simulink model "UNIFIER"  (R2023b)
settings: Solver=ode1  StartTime=0.0  StopTime=194  FixedStep=1/500  RelTol=1e-3
values from neighbouring files (symbols this model uses):
  b = 20.11467    [UNIFIERLanding_20240613_190735.mat]    (also in UNIFIER_LOAD.m; UNIFIER_LOADsim.m; UNIFIER_trim_out_20240612_032607.mat)
  c = 1.43676    [UNIFIERLanding_20240613_190735.mat]    (also in UNIFIER_LOAD.m; UNIFIER_LOADsim.m; UNIFIER_trim_out_20240612_032607.mat)
  DEP_INTEG_IC = 117.49388    [UNIFIER_LOAD.m]    (also in UNIFIER_LOADsim.m; UNIFIER_trim_out_20240612_032607.mat)
  dp_DEP =     [UNIFIERLanding_20240613_190735.mat]    (also in UNIFIER_trim_out_20240612_032607.mat)
  dp_FUSE_FIN =     [UNIFIER_trim_out_20240612_032607.mat]
  dp_HTU =     [UNIFIERLanding_20240613_190735.mat]    (also in UNIFIER_trim_out_20240612_032607.mat)
  dp_VTAIL =     [UNIFIER_trim_out_20240612_032607.mat]
  dp_VTAIL_INDUCED =     [UNIFIER_trim_out_20240612_032607.mat]
  dp_WING_root =     [UNIFIER_trim_out_20240612_032607.mat]
  dp_WING_tip =     [UNIFIER_trim_out_20240612_032607.mat]
  dumax = [1.0471975512 1.0471975512 1.0471975512 0.174532925199 2 2 2]    [UNIFIERLanding_20240613_190735.mat]
  Euler0 = xstar(7:9)'    [UNIFIER_6DOFsim_init.m]    (also in UNIFIER_LOAD.m = [0, 0, 0]; UNIFIER_LOADsim.m = [0, 0, 0]; UNIFIER_trim_out_20240612_032607.mat = [3.43106170069e-06 0.0515008506278 -2.79252663434])
  ground_alt = 0    [UNIFIER_LOAD.m]    (also in UNIFIER_LOADsim.m; UNIFIER_trim_out_20240612_032607.mat)
  m = 7057    [UNIFIERLanding_20240613_190735.mat]    (also in UNIFIER_LOAD.m; UNIFIER_LOADsim.m; UNIFIER_trim_out_20240612_032607.mat)
  omegab0 = xstar(10:12)'    [UNIFIER_6DOFsim_init.m]    (also in UNIFIER_LOAD.m = [0,0,0]; UNIFIER_LOADsim.m = [0,0,0]; UNIFIER_trim_out_20240612_032607.mat = [0 0 0])
  S = 29.98388    [UNIFIERLanding_20240613_190735.mat]    (also in UNIFIER_LOAD.m; UNIFIER_LOADsim.m; UNIFIER_trim_out_20240612_032607.mat)
  sensor_delay_steps = 5    [UNIFIER_LOAD.m]    (also in UNIFIER_LOADsim.m; UNIFIER_trim_out_20240612_032607.mat)
  solution =     [UNIFIERLanding_20240613_190735.mat]
  u1_0 = [ustar(1), -1*ustar(1), ustar(3)-ustar(2), ustar(3)+ustar(2), ustar(4), ustar(4)]    [UNIFIER_6DOFsim_init.m]    (also in UNIFIER_LOAD.m = [2.1112539e-05, -2.1112539e-05, -0.085004635, -0.084972650, ; UNIFIER_LOADsim.m = [2.1112539e-05, -2.1112539e-05, -0.085004635, -0.084972650, ; UNIFIER_trim_out_20240612_032607.mat = [2.1112539e-05 -2.1112539e-05 -0.085004635 -0.08497265 0.197)
  u2_0 = ones(1,12) .* ustar(5)    [UNIFIER_6DOFsim_init.m]    (also in UNIFIER_LOAD.m = ones(1,12) .* 0.4252; UNIFIER_LOADsim.m = ones(1,12) .* 0.4252; UNIFIER_trim_out_20240612_032607.mat = [0.4252 0.4252 0.4252 0.4252 0.4252 0.4252 0.4252 0.4252 0.4)
  u3_0 = ustar(7)    [UNIFIER_6DOFsim_init.m]    (also in UNIFIER_LOAD.m = 0.089689; UNIFIER_LOADsim.m = 0.089689; UNIFIER_trim_out_20240612_032607.mat = 0.089689)
  u4_0 = 0    [UNIFIER_6DOFsim_init.m]    (also in UNIFIER_LOAD.m; UNIFIER_LOADsim.m; UNIFIER_trim_out_20240612_032607.mat)
  u_trim = ustar    [UNIFIER_6DOFsim_init.m]    (also in UNIFIER_LOAD.m = [0.0; UNIFIER_LOADsim.m = [0.0)
  umax = [0.436332312999 0.523598775598 0.523598775598 0.436332312999 1 1 1]    [UNIFIERLanding_20240613_190735.mat]    (also in UNIFIER_trim_out_20240612_032607.mat)
  umin = [-0.436332312999 -0.523598775598 -0.523598775598 0 0 -1 -0.5]    [UNIFIERLanding_20240613_190735.mat]    (also in UNIFIER_trim_out_20240612_032607.mat)
  Va = [72.7399985115 72.2978466179 70.3592089076 68.5755686022 67.5674222915 66.8967003826 65.8958642605 64.4243196248 62.667507398 61.0171213882 59.8601734245 59.2796795419 ... (250 elements, 250x1)]    [UNIFIERLanding_20240613_190735.mat]
  Vb0 = xstar(4:6)'    [UNIFIER_6DOFsim_init.m]    (also in UNIFIER_LOAD.m = [72.731047032614440, 0, 1.142307104518741]; UNIFIER_LOADsim.m = [72.731047032614440, 0, 1.142307104518741]; UNIFIER_trim_out_20240612_032607.mat = [52.6789583502 0 2.71559652634])
  vtail_dist_to_wing = 7.8070    (= 7.807)    [UNIFIER_LOAD.m]    (also in UNIFIER_LOADsim.m; UNIFIER_trim_out_20240612_032607.mat)
  vtail_nodes = [dp_VTAIL.Xs_LE;     dp_VTAIL.Ys_LE;     dp_VTAIL.Zs_LE]    [UNIFIER_LOAD.m]    (also in UNIFIER_LOADsim.m; UNIFIER_trim_out_20240612_032607.mat = [-16.4894695282 -2.83441376686 -2.73765826225 -16.1370849609)
  wing_nodes = [fliplr(dp_WING_tip.LE_Xs),fliplr(dp_WING_root.LE_Xs),dp_WING_root.LE_Xs,dp_WING_tip.LE_Xs;     fliplr(-dp_WING_tip.LE_Ys),fliplr(-dp_WING_root.LE_Ys),dp_WING_root.LE_Ys,dp_WING_tip.LE_Ys;     fliplr(dp_WING_tip.LE_Zs),fliplr(dp_WING_root.LE_Zs),dp_WING_root.LE_Zs,dp_WING_tip.LE_Zs]    [UNIFIER_LOAD.m]    (also in UNIFIER_LOADsim.m; UNIFIER_trim_out_20240612_032607.mat = [-7.70795631409 -9.67500019073 -0.98178178072 -7.66801691055)
  Xe0 = xstar(1:3)'    [UNIFIER_6DOFsim_init.m]    (also in UNIFIER_LOAD.m = [0,0,-1219]; UNIFIER_LOADsim.m = [0,0,-1219]; UNIFIER_trim_out_20240612_032607.mat = [0 0 -1100])
  xyz_cg = [-8.09 0 -0.2]    [UNIFIERLanding_20240613_190735.mat]    (also in UNIFIER_LOAD.m = [-8.09,0,-0.2]; UNIFIER_LOADsim.m = [-8.09,0,-0.2]; UNIFIER_trim_out_20240612_032607.mat)
  xyz_DEP = [-6.9629998 -10.05 -0.90899998 -6.921 -8.4499998 -0.792 -6.8660002 -6.8499999 -0.82300001 -6.8099999 -5.25 -0.85000002 ... (36 elements, 3x12)]    [UNIFIERLanding_20240613_190735.mat]    (also in UNIFIER_LOAD.m = [ -6.9629998	-6.9210000	-6.8660002	-6.8099999	-6.7540002	-6.; UNIFIER_LOADsim.m = [ -6.9629998	-6.9210000	-6.8660002	-6.8099999	-6.7540002	-6.; UNIFIER_trim_out_20240612_032607.mat)
undefined symbols (not defined in the file or in its folder): Earth, F, MIL, WGS84
libraries: simulink_extras x23, aerolibactuator x16, dspnetwork x15, sharedutil x14, sharedtransform x7, aerolibtransform2 x5, slpidlib x5, simulink x5, aerolibwind2 x4, matrix_library x1, shared6dof x1, aerolibatmos2 x1
(part 4 of 6)

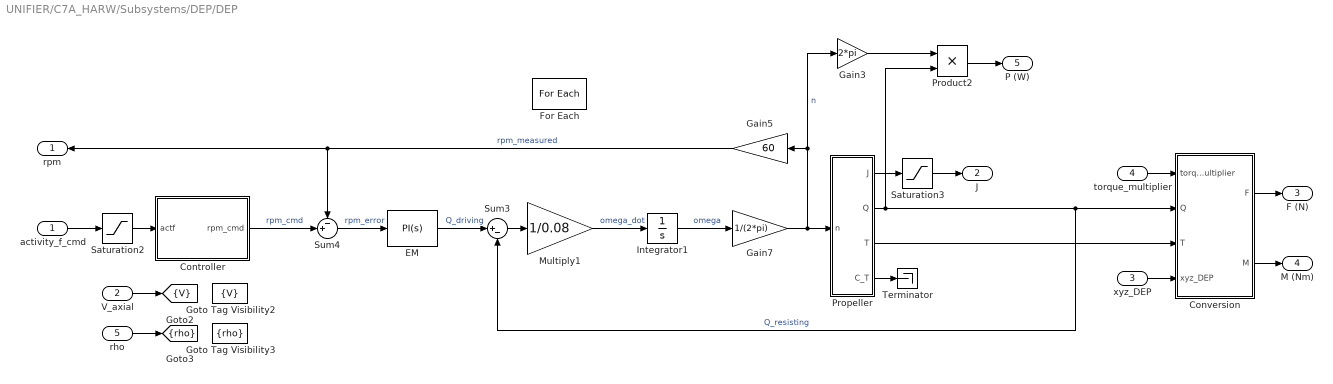
== system UNIFIER/C7A_HARW/Subsystems/DEP/DEP ==
  activity_f_cmd : Inport  Partition=on  PartitionDimension=1  PartitionWidth=1  PartitionOffset=0
  V_axial : Inport  Port=2  Partition=on  PartitionDimension=1  PartitionWidth=1  PartitionOffset=0
  xyz_DEP : Inport  Port=3  Partition=on  PartitionDimension=2  PartitionWidth=1  PartitionOffset=0
  torque_multiplier : Inport  Port=4  Partition=on  PartitionDimension=1  PartitionWidth=1  PartitionOffset=0
  rho : Inport  Port=5
  Controller : Subsystem
  Conversion : Subsystem
  EM : slpidlib/PID Controller  Controller=PI  Form=Parallel  TimeDomain=Continuous-time  UseExternalTs=off  SampleTime=-1  IntegratorMethod=Forward Euler  FilterMethod=Forward Euler  ControllerParametersSource=internal  P=0.768856317292492  I=33.2713838828509  UseKiTs=off  D=0  N=100  UseFilter=on  TunerSelectOption=Transfer Function Based (PID Tuner App)  InitialConditionSource=internal  InitialConditionForIntegrator=DEP_PID_IC  InitialConditionForFilter=0  DifferentiatorICPrevScaledInput=0  ExternalReset=none  TrackingMode=off  Kt=1  LimitOutput=on  SatLimitsSource=internal  UpperSaturationLimit=284  LowerSaturationLimit=-284  LinearizeAsGain=on  AntiWindupMode=clamping  Kb=1  LimitIntegrator=off  UpperIntegratorSaturationLimit=inf  LowerIntegratorSaturationLimit=-inf  POutMin=[]  POutMax=[]  IOutMin=[]  IOutMax=[]  DOutMin=[]  DOutMax=[]  NOutMin=[]  NOutMax=[]  SumOutMin=[]  SumOutMax=[]  SaturationOutMin=[]  SaturationOutMax=[]  PParamMin=[]  PParamMax=[]  IParamMin=[]  IParamMax=[]  DParamMin=[]  DParamMax=[]  NParamMin=[]  NParamMax=[]  KbParamMin=[]  KbParamMax=[]  KtParamMin=[]  KtParamMax=[]  KbOutMin=[]  KbOutMax=[]  KtOutMin=[]  KtOutMax=[]  IntegratorOutMin=[]  IntegratorOutMax=[]  FilterOutMin=[]  FilterOutMax=[]  SumI1OutMin=[]  SumI1OutMax=[]  SumI2OutMin=[]  SumI2OutMax=[]  SumI3OutMin=[]  SumI3OutMax=[]  SumI4OutMin=[]  SumI4OutMax=[]  SumDOutMin=[]  SumDOutMax=[]  DifferentiatorOutMin=[]  DifferentiatorOutMax=[]  FilterDiffOutCoefMin=[]  FilterDiffOutCoefMax=[]  ReciprocalOutMin=[]  ReciprocalOutMax=[]  SumDenOutMin=[]  SumDenOutMax=[]  SumNumOutMin=[]  SumNumOutMax=[]  DivideOutMin=[]  DivideOutMax=[]  UdiffTsProdOutMin=[]  UdiffTsProdOutMax=[]  NTsProdOutMin=[]  NTsProdOutMax=[]  UintegralTsProdOutMin=[]  UintegralTsProdOutMax=[]  UngainTsProdOutMin=[]  UngainTsProdOutMax=[]  ClampingZeroOutDataTypeStr=Inherit: Inherit via back propagation  ClampingZeroOutMin=[]  ClampingZeroOutMax=[]  FilterDenConstantOutDataTypeStr=Inherit: Inherit via back propagation  FilterDenConstantOutMin=[]  FilterDenConstantOutMax=[]  PCopyOutDataTypeStr=Inherit: Inherit via back propagation  PCopyOutMin=[]  PCopyOutMax=[]  NCopyOutDataTypeStr=Inherit: Inherit via back propagation  NCopyOutMin=[]  NCopyOutMax=[]  IntegratorContinuousStateAttributes=''  IntegratorStateMustResolveToSignalObject=off  IntegratorRTWStateStorageClass=Auto  FilterContinuousStateAttributes=''  FilterStateMustResolveToSignalObject=off  FilterRTWStateStorageClass=Auto  ParallelPVariant=InternalParameters  IdealPVariant=Disabled  IVariant=InternalParameters  DVariant=Disabled  IntegratorVariant=Continuous  SatVariant=Enabled  AWVariant=ContClampingParallel  PCopyVariant=Disabled  TRVariant=Disabled  FdbkBlocksVariant=Forward  IdealPFdbkVariant=Disabled  SatFdbkVariant=Disabled  DerivativeFilterVariant=Disabled  NVariant=Disabled  NCopyVariant=Disabled_SignalSpec  FilterICVariant=Disabled  IntegratorICVariant=InternalICs  ExternalResetVariant=Disabled  TRSumVariant=Passthrough  SumFdbkVariant=Disabled  SumVariant=Sum_PI  TsampFilterVariant=InternalTs  TsampNgainVariant=Passthrough  TsampIntegralVariant=Disabled_SignalSpec  ExternalSaturationOutDataTypeStr=Inherit: Same as second input
  For Each : ForEach  DisableCoverage=on  SpecifiedNumIters=12
  Gain3 : Gain  Gain=2*pi
  Gain5 : Gain  Gain=60
  Gain7 : Gain  Gain=1/(2*pi)
  Goto Tag Visibility2 : GotoTagVisibility  GotoTag=V
  Goto Tag Visibility3 : GotoTagVisibility  GotoTag=rho
  Integrator1 : Integrator  InitialCondition=DEP_INTEG_IC
  Multiply1 : Gain  Gain=1/0.08
  Product2 : Product
  Propeller : Subsystem
  Saturation2 : Saturate  UpperLimit=1  LowerLimit=0
  Saturation3 : Saturate  UpperLimit=5  LowerLimit=0.2
  Sum3 : Sum  Inputs=|+-
  Sum4 : Sum  Inputs=-+|
  Terminator : Terminator
  rpm : Outport  ConcatenationDimension=1
  J : Outport  Port=2  ConcatenationDimension=1
  F (N) : Outport  Port=3  ConcatenationDimension=2
  M (Nm) : Outport  Port=4  ConcatenationDimension=2
  P (W) : Outport  Port=5  ConcatenationDimension=1
  tag scope: V=scoped, rho=scoped
  wires:
  Conversion/1(F) -> F (N)/1
  Conversion/2(M) -> M (Nm)/1
  Saturation3/1 -> J/1
  Propeller/4(C_T) -> Terminator/1
  activity_f_cmd/1 -> Saturation2/1
  Propeller/1(J) -> Saturation3/1
  Controller/1(rpm_cmd) -> Sum4/2  "rpm_cmd"
  Gain3/1 -> Product2/1
  xyz_DEP/1 -> Conversion/4(xyz_DEP)
  Multiply1/1 -> Integrator1/1  "omega_dot"
  Sum4/1 -> EM/1  "rpm_error"
  Gain7/1 -> Gain3/1, Gain5/1, Propeller/1(n)  "n"
  EM/1 -> Sum3/1  "Q_driving"
  V_axial/1 -> [V]
  Product2/1 -> P (W)/1
  torque_multiplier/1 -> Conversion/1(torque_multiplier)
  Gain5/1 -> rpm/1, Sum4/1  "rpm_measured"
  Propeller/3(T) -> Conversion/3(T)
  rho/1 -> [rho]
  Propeller/2(Q) -> Product2/2, Conversion/2(Q), Sum3/2  "Q_resisting"
  Saturation2/1 -> Controller/1(actf)
  Sum3/1 -> Multiply1/1
  Integrator1/1 -> Gain7/1  "omega"

== system UNIFIER/C7A_HARW/Subsystems/HTU/PropAndMotor ==
  Vrw_mag_eas : Inport
  T_cmd (N) : Inport  Port=2
  1-D Lookup Table : Lookup_n-D  NumberOfTableDimensions=1  BreakpointsForDimension1=dp_HTU.limits.V_low_lim  IndexSearchMethod=Linear search  BeginIndexSearchUsingPreviousIndexResult=on  Table=dp_HTU.limits.T_low_lim  InternalRulePriority=Speed  RndMeth=Simplest
  1-D Lookup Table1 : Lookup_n-D  NumberOfTableDimensions=1  BreakpointsForDimension1=dp_HTU.limits.V_up_lim  IndexSearchMethod=Linear search  BeginIndexSearchUsingPreviousIndexResult=on  Table=dp_HTU.limits.T_up_lim  InternalRulePriority=Speed  RndMeth=Simplest
  Linear Second-Order Actuator : aerolibactuator/Linear Second-Order Actuator  wn_fin=8  z_fin=1.1  fin_act_0=0  fin_act_vel=0
  P lookup : Lookup_n-D  BreakpointsForDimension1=dp_HTU.V_vec  BreakpointsForDimension2=dp_HTU.T_vec  IndexSearchMethod=Linear search  BeginIndexSearchUsingPreviousIndexResult=on  Table=dp_HTU.P_grid  InternalRulePriority=Speed  RndMeth=Simplest
      settings: InputPortMap=u0,u1
  Saturation Dynamic : simulink/Discontinuities/Saturation Dynamic  OutMin=[]  OutMax=[]  OutDataTypeStr=Inherit: Same as second input  OutDataType=fixdt(1, 16)  OutScaling=2^-10  DoSatur=off
  P (kW) : Outport
  T (N) : Outport  Port=2
  wires:
  Vrw_mag_eas/1 -> P lookup/1, 1-D Lookup Table/1, 1-D Lookup Table1/1
  Saturation Dynamic/1 -> Linear Second-Order Actuator/1
  P lookup/1 -> P (kW)/1
  1-D Lookup Table1/1 -> Saturation Dynamic/1
  1-D Lookup Table/1 -> Saturation Dynamic/3
  T_cmd (N)/1 -> Saturation Dynamic/2
  Linear Second-Order Actuator/1 -> T (N)/1, P lookup/2

== system UNIFIER/C7A_HARW/Subsystems/LandingGears/LeftMain ==
  xyz_gear : Inport  PortDimensions=3
  Euler : Inport  Port=2  PortDimensions=3
  X_e : Inport  Port=3  PortDimensions=3
  ground_alt : Inport  Port=4
  omega : Inport  Port=5
  V_b : Inport  Port=6  PortDimensions=3
  DetermineGroundImpact : Subsystem
  FrameTransfer : Subsystem
  GearForceSystem : Subsystem
      settings: PortSchema="{\"entries\":[{\"content\":{\"sides\":[{\"content\":{\"connectorIds\":[\"In1\",\"In2\"]},\"type\":\"ConnectorPlacement.EquallySpacedRectSide\",\"uuid\":\"d290905f-60cf-4bc0-bab1-4e61329254ed\"},{\"content\":{\"connectorIds\":[\"Out1\"],\"side\":\"RIGHT\"},\"type\":\"ConnectorPlacement.EquallySpacedRectSide\",\"uuid\":\"8978d452-e293-46ff-9875-eaa6c076b0ed\"},{\"content\":{\"connectorIds\":[\"In3\"],\"side\":\"TOP\"},\"type\":\"ConnectorPlacement.EquallySpacedRectSide\",\"uuid\":\"a7915404-bc15-4a50-b2f6-71702d493273\"},{\"content\":{\"connectorIds\":[],\"side\":\"HIDDEN\"},\"type\":\"ConnectorPlacement.EquallySpacedRectSide\",\"uuid\":\"71da3c07-875d-44a9-a817-88149ba8aea4\"}]},\"type\":\"ConnectorPlacement.EquallySpacedConnector\",\"uuid\":\"ffb36ab3-c4a0-4dd1-8d55-bd9c51a110f4\"}],\"packageUris\":[\"http://schema.mathworks.com/mf0/Connector/R2020b\"],\"version\":\"1.0\"}"
  GetDeflection : Subsystem
  PointAndVelocityTransformation : Subsystem
  Scope : Scope
  Scope1 : Scope
  Scope3 : Scope
  F : Outport
  M : Outport  Port=2
  impact_flag : Outport  Port=3
  wires:
  DetermineGroundImpact/1(dz_to_ground) -> Scope/1
  ground_alt/1 -> DetermineGroundImpact/2(ground_alt)
  GetDeflection/1(dz) -> GearForceSystem/2(dz)
  PointAndVelocityTransformation/1(X_gear) -> GetDeflection/2(X_tip), DetermineGroundImpact/1(X_gear)
  GearForceSystem/1(F_gear_total) -> Scope1/1, FrameTransfer/2(F_gear_total)
  omega/1 -> PointAndVelocityTransformation/4(omega)
  xyz_gear/1 -> PointAndVelocityTransformation/1(xyz_gear), FrameTransfer/1(xyz_shock_absorber)
  FrameTransfer/2(M_b) -> M/1
  DetermineGroundImpact/2(impact_flag) -> impact_flag/1, GearForceSystem/3(impact_flag), Scope3/1
  V_b/1 -> PointAndVelocityTransformation/5(V_b)
  FrameTransfer/1(F_b) -> F/1
  DetermineGroundImpact/3(X_impact) -> GetDeflection/1(X_impact)
  PointAndVelocityTransformation/2(V_gear) -> GearForceSystem/1(V_gear)
  X_e/1 -> PointAndVelocityTransformation/2(X_e)
  Euler/1 -> PointAndVelocityTransformation/3(Euler)

== system UNIFIER/C7A_HARW/Subsystems/LandingGears/Nose ==
  xyz_gear : Inport  PortDimensions=3
  Euler : Inport  Port=2  PortDimensions=3
  X_e : Inport  Port=3  PortDimensions=3
  ground_alt : Inport  Port=4
  omega : Inport  Port=5
  V_b : Inport  Port=6  PortDimensions=3
  DetermineGroundImpact : Subsystem
  FrameTransfer : Subsystem
  GearForceSystem : Subsystem
      settings: PortSchema="{\"entries\":[{\"content\":{\"sides\":[{\"content\":{\"connectorIds\":[\"In1\",\"In2\"]},\"type\":\"ConnectorPlacement.EquallySpacedRectSide\",\"uuid\":\"d290905f-60cf-4bc0-bab1-4e61329254ed\"},{\"content\":{\"connectorIds\":[\"Out1\"],\"side\":\"RIGHT\"},\"type\":\"ConnectorPlacement.EquallySpacedRectSide\",\"uuid\":\"8978d452-e293-46ff-9875-eaa6c076b0ed\"},{\"content\":{\"connectorIds\":[\"In3\"],\"side\":\"TOP\"},\"type\":\"ConnectorPlacement.EquallySpacedRectSide\",\"uuid\":\"a7915404-bc15-4a50-b2f6-71702d493273\"},{\"content\":{\"connectorIds\":[],\"side\":\"HIDDEN\"},\"type\":\"ConnectorPlacement.EquallySpacedRectSide\",\"uuid\":\"71da3c07-875d-44a9-a817-88149ba8aea4\"}]},\"type\":\"ConnectorPlacement.EquallySpacedConnector\",\"uuid\":\"ffb36ab3-c4a0-4dd1-8d55-bd9c51a110f4\"}],\"packageUris\":[\"http://schema.mathworks.com/mf0/Connector/R2020b\"],\"version\":\"1.0\"}"
  GetDeflection : Subsystem
  PointAndVelocityTransformation : Subsystem
  Scope : Scope
  Scope1 : Scope
  Scope3 : Scope
  F : Outport
  M : Outport  Port=2
  impact_flag : Outport  Port=3
  wires:
  DetermineGroundImpact/1(dz_to_ground) -> Scope/1
  ground_alt/1 -> DetermineGroundImpact/2(ground_alt)
  GetDeflection/1(dz) -> GearForceSystem/2(dz)
  PointAndVelocityTransformation/1(X_gear) -> GetDeflection/2(X_tip), DetermineGroundImpact/1(X_gear)
  GearForceSystem/1(F_gear_total) -> Scope1/1, FrameTransfer/2(F_gear_total)
  omega/1 -> PointAndVelocityTransformation/4(omega)
  xyz_gear/1 -> PointAndVelocityTransformation/1(xyz_gear), FrameTransfer/1(xyz_shock_absorber)
  FrameTransfer/2(M_b) -> M/1
  DetermineGroundImpact/2(impact_flag) -> impact_flag/1, GearForceSystem/3(impact_flag), Scope3/1
  V_b/1 -> PointAndVelocityTransformation/5(V_b)
  FrameTransfer/1(F_b) -> F/1
  DetermineGroundImpact/3(X_impact) -> GetDeflection/1(X_impact)
  PointAndVelocityTransformation/2(V_gear) -> GearForceSystem/1(V_gear)
  X_e/1 -> PointAndVelocityTransformation/2(X_e)
  Euler/1 -> PointAndVelocityTransformation/3(Euler)

== system UNIFIER/C7A_HARW/Subsystems/LandingGears/RightMain ==
  xyz_gear : Inport  PortDimensions=3
  Euler : Inport  Port=2  PortDimensions=3
  X_e : Inport  Port=3  PortDimensions=3
  ground_alt : Inport  Port=4
  omega : Inport  Port=5
  V_b : Inport  Port=6  PortDimensions=3
  DetermineGroundImpact : Subsystem
  FrameTransfer : Subsystem
  GearForceSystem : Subsystem
      settings: PortSchema="{\"entries\":[{\"content\":{\"sides\":[{\"content\":{\"connectorIds\":[\"In1\",\"In2\"]},\"type\":\"ConnectorPlacement.EquallySpacedRectSide\",\"uuid\":\"d290905f-60cf-4bc0-bab1-4e61329254ed\"},{\"content\":{\"connectorIds\":[\"Out1\"],\"side\":\"RIGHT\"},\"type\":\"ConnectorPlacement.EquallySpacedRectSide\",\"uuid\":\"8978d452-e293-46ff-9875-eaa6c076b0ed\"},{\"content\":{\"connectorIds\":[\"In3\"],\"side\":\"TOP\"},\"type\":\"ConnectorPlacement.EquallySpacedRectSide\",\"uuid\":\"a7915404-bc15-4a50-b2f6-71702d493273\"},{\"content\":{\"connectorIds\":[],\"side\":\"HIDDEN\"},\"type\":\"ConnectorPlacement.EquallySpacedRectSide\",\"uuid\":\"71da3c07-875d-44a9-a817-88149ba8aea4\"}]},\"type\":\"ConnectorPlacement.EquallySpacedConnector\",\"uuid\":\"ffb36ab3-c4a0-4dd1-8d55-bd9c51a110f4\"}],\"packageUris\":[\"http://schema.mathworks.com/mf0/Connector/R2020b\"],\"version\":\"1.0\"}"
  GetDeflection : Subsystem
  PointAndVelocityTransformation : Subsystem
  Scope : Scope
  Scope1 : Scope
  Scope3 : Scope
  F : Outport
  M : Outport  Port=2
  impact_flag : Outport  Port=3
  wires:
  DetermineGroundImpact/1(dz_to_ground) -> Scope/1
  ground_alt/1 -> DetermineGroundImpact/2(ground_alt)
  GetDeflection/1(dz) -> GearForceSystem/2(dz)
  PointAndVelocityTransformation/1(X_gear) -> GetDeflection/2(X_tip), DetermineGroundImpact/1(X_gear)
  GearForceSystem/1(F_gear_total) -> Scope1/1, FrameTransfer/2(F_gear_total)
  omega/1 -> PointAndVelocityTransformation/4(omega)
  xyz_gear/1 -> PointAndVelocityTransformation/1(xyz_gear), FrameTransfer/1(xyz_shock_absorber)
  FrameTransfer/2(M_b) -> M/1
  DetermineGroundImpact/2(impact_flag) -> impact_flag/1, GearForceSystem/3(impact_flag), Scope3/1
  V_b/1 -> PointAndVelocityTransformation/5(V_b)
  FrameTransfer/1(F_b) -> F/1
  DetermineGroundImpact/3(X_impact) -> GetDeflection/1(X_impact)
  PointAndVelocityTransformation/2(V_gear) -> GearForceSystem/1(V_gear)
  X_e/1 -> PointAndVelocityTransformation/2(X_e)
  Euler/1 -> PointAndVelocityTransformation/3(Euler)

== system UNIFIER/C7A_HARW/Subsystems/LandingGears/SideForceAndSteeringAndBraking ==
  impact_flag_main : Inport
  impact_flag_nose : Inport  Port=2
  V_b : Inport  Port=3  PortDimensions=3
  Fz_main : Inport  Port=4
  Fz_nose : Inport  Port=5
  sidestick_bus : Inport  Port=6
  Bus Selector : BusSelector  OutputSignals=yaw_raw,buttons
  Constant1 : Constant  Value=[-8.8,0,2]
  Constant2 : Constant  Value=[-1.3,0,1.9]
  ForceSystem : Subsystem
  FrameTransfer1 : Subsystem
  FrameTransfer2 : Subsystem
  Sum : Sum  Inputs=|++
  Sum1 : Sum  Inputs=|++
  F_b : Outport
  M_b : Outport  Port=2
  wires:
  impact_flag_main/1 -> ForceSystem/1(impact_flag_main)
  V_b/1 -> ForceSystem/3(V_b)
  ForceSystem/1(F_main_gear) -> FrameTransfer1/2(F_total)
  Fz_main/1 -> ForceSystem/4(Fz_main)
  Constant1/1 -> FrameTransfer1/1(xyz)
  FrameTransfer1/1(F_b) -> Sum/1
  FrameTransfer1/2(M_b) -> Sum1/1
  Fz_nose/1 -> ForceSystem/5(Fz_nose)
  impact_flag_nose/1 -> ForceSystem/2(impact_flag_nose)
  sidestick_bus/1 -> Bus Selector/1
  Bus Selector/1 -> ForceSystem/6(yaw_raw)  "<yaw_raw>"
  Bus Selector/2 -> ForceSystem/7(buttons)  "<buttons>"
  ForceSystem/2(F_nose_gear) -> FrameTransfer2/2(F_total)
  Constant2/1 -> FrameTransfer2/1(xyz)
  Sum/1 -> F_b/1
  Sum1/1 -> M_b/1
  FrameTransfer2/1(F_b) -> Sum/2
  FrameTransfer2/2(M_b) -> Sum1/2

== system UNIFIER/PACER/soft real time subsystem/get elapsed wall-clock time/triggered capture & hold ==
  note: Marc Compere
      | comperem@gmail.com
      | created  : 13 September 2002
      | modified: 24 February 2004
  note: if trigger==1,
      |    out(k) = value_to_capture(k)
      | else,
      |    out(k) = out(k-1)
  value to capture : Inport
  trigger : Inport  Port=2
  . : UnitDelay  SampleTime=-1  HasFrameUpgradeWarning=on
  Relational Operator : RelationalOperator  Operator===  InputSameDT=off
  Switch : Switch  Threshold=0.5  InputSameDT=off
  const : Constant
  out : Outport
  wires:
  trigger/1 -> Relational Operator/1
  const/1 -> Relational Operator/2
  Relational Operator/1 -> Switch/2
  Switch/1 -> ./1, out/1  "out(k)"
  value to capture/1 -> Switch/1
  ./1 -> Switch/3  "out(k-1)"

== system UNIFIER/C7A_HARW/Aero/FinFuselageForces/Subsystem1/Subsystem ==
  beta : Inport
  alpha : Inport  Port=2
  Prelookup : PreLookup  BreakpointsData=dp_FUSE_FIN.beta  IndexSearchMethod=Linear search  BeginIndexSearchUsingPreviousIndexResult=on  ExtrapMethod=Linear
  Prelookup1 : PreLookup  BreakpointsData=dp_FUSE_FIN.aoa  IndexSearchMethod=Linear search  BeginIndexSearchUsingPreviousIndexResult=on  ExtrapMethod=Linear
  Out1 : Outport
  Out2 : Outport  Port=2
  Out3 : Outport  Port=3
  Out4 : Outport  Port=4
  wires:
  Prelookup/1 -> Out1/1
  alpha/1 -> Prelookup1/1
  beta/1 -> Prelookup/1
  Prelookup1/1 -> Out3/1
  Prelookup1/2 -> Out4/1
  Prelookup/2 -> Out2/1

== system UNIFIER/C7A_HARW/Aero/VtailForces/Subsystem/CrossProduct1 ==
  r : Inport  Partition=on  PartitionDimension=2  PartitionWidth=1  PartitionOffset=0
  F : Inport  Port=2  Partition=on  PartitionDimension=2  PartitionWidth=1  PartitionOffset=0
  3x3 Cross Product : sharedutil/3x3 Cross Product  aMode=aMode
  CG : Constant  Value=xyz_cg
  Cast : DataTypeConversion  OutDataTypeStr=single  SaturateOnIntegerOverflow=off  RndMeth=Floor
  For Each : ForEach  DisableCoverage=on  SpecifiedNumIters=16
  Minus : Sum  Inputs=+-
  M : Outport  ConcatenationDimension=2
  wires:
  F/1 -> 3x3 Cross Product/2
  r/1 -> Minus/1
  3x3 Cross Product/1 -> M/1
  CG/1 -> Cast/1
  Minus/1 -> 3x3 Cross Product/1
  Cast/1 -> Minus/2

== system UNIFIER/C7A_HARW/Aero/VtailForces/VtailForces/WingRootPreLookup ==
  rude_defl_nodes : Inport
  alpha_nodes : Inport  Port=2
  beta_nodes : Inport  Port=3
  Constant8 : Constant  Value=0:15
  Prelookup : PreLookup  BreakpointsData=dp_VTAIL.rude_defl  IndexSearchMethod=Linear search  BeginIndexSearchUsingPreviousIndexResult=on  ExtrapMethod=Linear
  Prelookup1 : PreLookup  BreakpointsData=dp_VTAIL.alphas  IndexSearchMethod=Linear search  BeginIndexSearchUsingPreviousIndexResult=on  ExtrapMethod=Linear
  Prelookup2 : PreLookup  BreakpointsData=dp_VTAIL.betas  IndexSearchMethod=Linear search  BeginIndexSearchUsingPreviousIndexResult=on  ExtrapMethod=Linear
  Out1 : Outport
  Out2 : Outport  Port=2
  Out3 : Outport  Port=3
  Out4 : Outport  Port=4
  Out6 : Outport  Port=5
  Out7 : Outport  Port=6
  Out5 : Outport  Port=7
  wires:
  Prelookup/1 -> Out1/1
  Constant8/1 -> Out5/1
  Prelookup1/2 -> Out4/1
  Prelookup/2 -> Out2/1
  alpha_nodes/1 -> Prelookup1/1
  Prelookup1/1 -> Out3/1
  rude_defl_nodes/1 -> Prelookup/1
  beta_nodes/1 -> Prelookup2/1
  Prelookup2/1 -> Out6/1
  Prelookup2/2 -> Out7/1

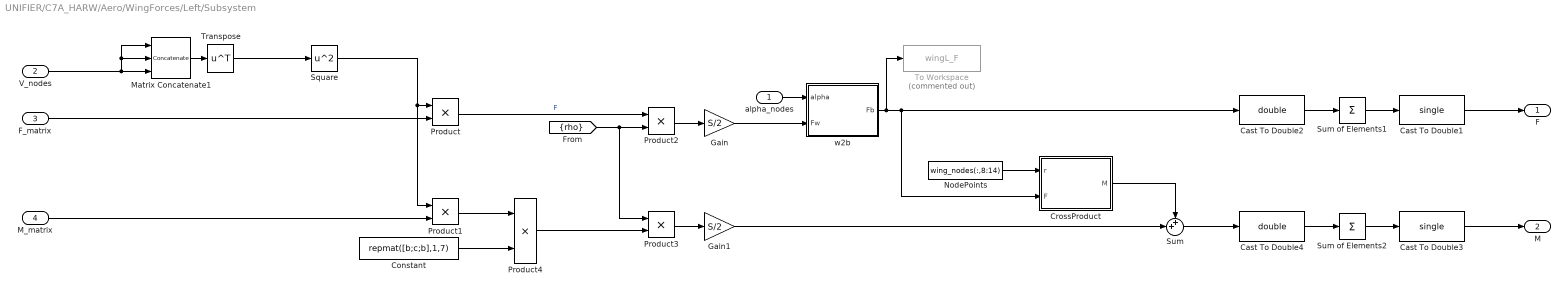
== system UNIFIER/C7A_HARW/Aero/WingForces/Left/Subsystem ==
  alpha_nodes : Inport
  V_nodes : Inport  Port=2
  F_matrix : Inport  Port=3
  M_matrix : Inport  Port=4
  Cast To Double1 : DataTypeConversion  OutDataTypeStr=single  SaturateOnIntegerOverflow=off  RndMeth=Floor
  Cast To Double2 : DataTypeConversion  OutDataTypeStr=double  SaturateOnIntegerOverflow=off  RndMeth=Floor
  Cast To Double3 : DataTypeConversion  OutDataTypeStr=single  SaturateOnIntegerOverflow=off  RndMeth=Floor
  Cast To Double4 : DataTypeConversion  OutDataTypeStr=double  SaturateOnIntegerOverflow=off  RndMeth=Floor
  Constant : Constant  Value=repmat([b;c;b],1,7)
  CrossProduct : Subsystem  TreatAsAtomicUnit=on
  Gain : Gain  Gain=S/2
  Gain1 : Gain  Gain=S/2
  Matrix Concatenate1 : Concatenate  NumInputs=3  Mode=Multidimensional array  ConcatenateDimension=2
  NodePoints : Constant  Value=wing_nodes(:,8:14)
  Product{,1..4} (5 alike) : Product
  Square : Math  Operator=square
  Sum : Sum  Inputs=++|
  Sum of Elements1 : Sum  Inputs=+  CollapseMode=Specified dimension  CollapseDim=2
  Sum of Elements2 : Sum  Inputs=+  CollapseMode=Specified dimension  CollapseDim=2
  To Workspace : ToWorkspace  Commented=on  VariableName=wingL_F  SaveFormat=Structure With Time  SampleTime=1/100
  Transpose : Math  Operator=transpose
  w2b : Subsystem  TreatAsAtomicUnit=on
  F : Outport
  M : Outport  Port=2
  wires:
  Product2/1 -> Gain/1
  F_matrix/1 -> Product/2
  [rho] -> Product3/1, Product2/2
  Product3/1 -> Gain1/1
  Constant/1 -> Product4/2
  Product4/1 -> Product3/2
  M_matrix/1 -> Product1/2
  Product1/1 -> Product4/1
  Gain1/1 -> Sum/2
  Product/1 -> Product2/1  "F"
  V_nodes/1 -> Matrix Concatenate1/1, Matrix Concatenate1/2, Matrix Concatenate1/3
  Transpose/1 -> Square/1
  Matrix Concatenate1/1 -> Transpose/1
  Square/1 -> Product1/1, Product/1
  w2b/1(Fb) -> To Workspace/1, Cast To Double2/1, CrossProduct/2(F)
  NodePoints/1 -> CrossProduct/1(r)
  CrossProduct/1(M) -> Sum/1
  Cast To Double1/1 -> F/1
  Gain/1 -> w2b/2(Fw)
  alpha_nodes/1 -> w2b/1(alpha)
  Cast To Double2/1 -> Sum of Elements1/1
  Sum of Elements1/1 -> Cast To Double1/1
  Sum of Elements2/1 -> Cast To Double3/1
  Cast To Double4/1 -> Sum of Elements2/1
  Sum/1 -> Cast To Double4/1
  Cast To Double3/1 -> M/1

== system UNIFIER/C7A_HARW/Aero/WingForces/Left/WingRootForces ==
  flap_defl : Inport
  alpha : Inport  Port=2
  V_node : Inport  Port=3
  DEP_J : Inport  Port=4
  Interpolation Using Prelookup1 : Interpolation_n-D  NumberOfTableDimensions=5  Table=dp_WING_root.CD  ExtrapMethod=Clip  ValidIndexMayReachLast=on  NumSelectionDims=1  InternalRulePriority=Speed  TableDataTypeStr=Inherit: Inherit from 'Table data'
      settings: InputPortMap=u0,u1,u2,u3,u4,u5,u6,u7,u8
  Interpolation Using Prelookup2 : Interpolation_n-D  NumberOfTableDimensions=5  Table=dp_WING_root.CS  ExtrapMethod=Clip  ValidIndexMayReachLast=on  NumSelectionDims=1  InternalRulePriority=Speed  TableDataTypeStr=Inherit: Inherit from 'Table data'
      settings: InputPortMap=u0,u1,u2,u3,u4,u5,u6,u7,u8
  Interpolation Using Prelookup3 : Interpolation_n-D  NumberOfTableDimensions=5  Table=dp_WING_root.CL  ExtrapMethod=Clip  ValidIndexMayReachLast=on  NumSelectionDims=1  InternalRulePriority=Speed  TableDataTypeStr=Inherit: Inherit from 'Table data'
      settings: InputPortMap=u0,u1,u2,u3,u4,u5,u6,u7,u8
  Interpolation Using Prelookup4 : Interpolation_n-D  NumberOfTableDimensions=5  Table=dp_WING_root.CMx  ExtrapMethod=Clip  ValidIndexMayReachLast=on  NumSelectionDims=1  InternalRulePriority=Speed  TableDataTypeStr=Inherit: Inherit from 'Table data'
      settings: InputPortMap=u0,u1,u2,u3,u4,u5,u6,u7,u8
  Interpolation Using Prelookup5 : Interpolation_n-D  NumberOfTableDimensions=5  Table=dp_WING_root.CMy  ExtrapMethod=Clip  ValidIndexMayReachLast=on  NumSelectionDims=1  InternalRulePriority=Speed  TableDataTypeStr=Inherit: Inherit from 'Table data'
      settings: InputPortMap=u0,u1,u2,u3,u4,u5,u6,u7,u8
  Interpolation Using Prelookup6 : Interpolation_n-D  NumberOfTableDimensions=5  Table=dp_WING_root.CMz  ExtrapMethod=Clip  ValidIndexMayReachLast=on  NumSelectionDims=1  InternalRulePriority=Speed  TableDataTypeStr=Inherit: Inherit from 'Table data'
      settings: InputPortMap=u0,u1,u2,u3,u4,u5,u6,u7,u8
  WingRootPreLookup : Subsystem
  CD : Outport
  CS : Outport  Port=2
  CL : Outport  Port=3
  CMx : Outport  Port=4
  CMy : Outport  Port=5
  CMz : Outport  Port=6
  wires:
  WingRootPreLookup/9(Out5) -> Interpolation Using Prelookup6/9, Interpolation Using Prelookup5/9, Interpolation Using Prelookup4/9, Interpolation Using Prelookup3/9, Interpolation Using Prelookup2/9, Interpolation Using Prelookup1/9
  WingRootPreLookup/3(Out3) -> Interpolation Using Prelookup6/3, Interpolation Using Prelookup5/3, Interpolation Using Prelookup4/3, Interpolation Using Prelookup3/3, Interpolation Using Prelookup2/3, Interpolation Using Prelookup1/3
  WingRootPreLookup/8(Out9) -> Interpolation Using Prelookup6/8, Interpolation Using Prelookup5/8, Interpolation Using Prelookup4/8, Interpolation Using Prelookup3/8, Interpolation Using Prelookup2/8, Interpolation Using Prelookup1/8
  WingRootPreLookup/1(Out1) -> Interpolation Using Prelookup6/1, Interpolation Using Prelookup5/1, Interpolation Using Prelookup4/1, Interpolation Using Prelookup3/1, Interpolation Using Prelookup2/1, Interpolation Using Prelookup1/1
  WingRootPreLookup/7(Out8) -> Interpolation Using Prelookup1/7, Interpolation Using Prelookup5/7, Interpolation Using Prelookup6/7, Interpolation Using Prelookup4/7, Interpolation Using Prelookup3/7, Interpolation Using Prelookup2/7
  flap_defl/1 -> WingRootPreLookup/1(flap_defl)
  WingRootPreLookup/4(Out4) -> Interpolation Using Prelookup6/4, Interpolation Using Prelookup5/4, Interpolation Using Prelookup4/4, Interpolation Using Prelookup3/4, Interpolation Using Prelookup2/4, Interpolation Using Prelookup1/4
  WingRootPreLookup/5(Out6) -> Interpolation Using Prelookup1/5, Interpolation Using Prelookup6/5, Interpolation Using Prelookup5/5, Interpolation Using Prelookup4/5, Interpolation Using Prelookup3/5, Interpolation Using Prelookup2/5
  Interpolation Using Prelookup1/1 -> CD/1
  WingRootPreLookup/6(Out7) -> Interpolation Using Prelookup6/6, Interpolation Using Prelookup5/6, Interpolation Using Prelookup4/6, Interpolation Using Prelookup3/6, Interpolation Using Prelookup2/6, Interpolation Using Prelookup1/6
  WingRootPreLookup/2(Out2) -> Interpolation Using Prelookup6/2, Interpolation Using Prelookup5/2, Interpolation Using Prelookup4/2, Interpolation Using Prelookup3/2, Interpolation Using Prelookup2/2, Interpolation Using Prelookup1/2
  DEP_J/1 -> WingRootPreLookup/4(DEP_J)
  V_node/1 -> WingRootPreLookup/3(V_node)
  alpha/1 -> WingRootPreLookup/2(alpha)
  Interpolation Using Prelookup2/1 -> CS/1
  Interpolation Using Prelookup3/1 -> CL/1
  Interpolation Using Prelookup4/1 -> CMx/1
  Interpolation Using Prelookup5/1 -> CMy/1
  Interpolation Using Prelookup6/1 -> CMz/1

== system UNIFIER/C7A_HARW/Aero/WingForces/Left/WingTipForces ==
  ail_defl : Inport
  alpha : Inport  Port=2
  V_node : Inport  Port=3
  DEP_J : Inport  Port=4
  Interpolation Using Prelookup1 : Interpolation_n-D  NumberOfTableDimensions=5  Table=dp_WING_tip.CD  ExtrapMethod=Clip  ValidIndexMayReachLast=on  NumSelectionDims=1  InternalRulePriority=Speed  TableDataTypeStr=Inherit: Inherit from 'Table data'
      settings: InputPortMap=u0,u1,u2,u3,u4,u5,u6,u7,u8
  Interpolation Using Prelookup2 : Interpolation_n-D  NumberOfTableDimensions=5  Table=dp_WING_tip.CS  ExtrapMethod=Clip  ValidIndexMayReachLast=on  NumSelectionDims=1  InternalRulePriority=Speed  TableDataTypeStr=Inherit: Inherit from 'Table data'
      settings: InputPortMap=u0,u1,u2,u3,u4,u5,u6,u7,u8
  Interpolation Using Prelookup3 : Interpolation_n-D  NumberOfTableDimensions=5  Table=dp_WING_tip.CL  ExtrapMethod=Clip  ValidIndexMayReachLast=on  NumSelectionDims=1  InternalRulePriority=Speed  TableDataTypeStr=Inherit: Inherit from 'Table data'
      settings: InputPortMap=u0,u1,u2,u3,u4,u5,u6,u7,u8
  Interpolation Using Prelookup4 : Interpolation_n-D  NumberOfTableDimensions=5  Table=dp_WING_tip.CMx  ExtrapMethod=Clip  ValidIndexMayReachLast=on  NumSelectionDims=1  InternalRulePriority=Speed  TableDataTypeStr=Inherit: Inherit from 'Table data'
      settings: InputPortMap=u0,u1,u2,u3,u4,u5,u6,u7,u8
  Interpolation Using Prelookup5 : Interpolation_n-D  NumberOfTableDimensions=5  Table=dp_WING_tip.CMy  ExtrapMethod=Clip  ValidIndexMayReachLast=on  NumSelectionDims=1  InternalRulePriority=Speed  TableDataTypeStr=Inherit: Inherit from 'Table data'
      settings: InputPortMap=u0,u1,u2,u3,u4,u5,u6,u7,u8
  Interpolation Using Prelookup6 : Interpolation_n-D  NumberOfTableDimensions=5  Table=dp_WING_tip.CMz  ExtrapMethod=Clip  ValidIndexMayReachLast=on  NumSelectionDims=1  InternalRulePriority=Speed  TableDataTypeStr=Inherit: Inherit from 'Table data'
      settings: InputPortMap=u0,u1,u2,u3,u4,u5,u6,u7,u8
  WingRootPreLookup : Subsystem
  CD : Outport
  CS : Outport  Port=2
  CL : Outport  Port=3
  CMx : Outport  Port=4
  CMy : Outport  Port=5
  CMz : Outport  Port=6
  wires:
  WingRootPreLookup/9(Out5) -> Interpolation Using Prelookup6/9, Interpolation Using Prelookup5/9, Interpolation Using Prelookup4/9, Interpolation Using Prelookup3/9, Interpolation Using Prelookup2/9, Interpolation Using Prelookup1/9
  WingRootPreLookup/3(Out3) -> Interpolation Using Prelookup6/3, Interpolation Using Prelookup5/3, Interpolation Using Prelookup4/3, Interpolation Using Prelookup3/3, Interpolation Using Prelookup2/3, Interpolation Using Prelookup1/3
  WingRootPreLookup/8(Out9) -> Interpolation Using Prelookup6/8, Interpolation Using Prelookup5/8, Interpolation Using Prelookup4/8, Interpolation Using Prelookup3/8, Interpolation Using Prelookup2/8, Interpolation Using Prelookup1/8
  WingRootPreLookup/1(Out1) -> Interpolation Using Prelookup6/1, Interpolation Using Prelookup5/1, Interpolation Using Prelookup4/1, Interpolation Using Prelookup3/1, Interpolation Using Prelookup2/1, Interpolation Using Prelookup1/1
  WingRootPreLookup/7(Out8) -> Interpolation Using Prelookup5/7, Interpolation Using Prelookup6/7, Interpolation Using Prelookup4/7, Interpolation Using Prelookup3/7, Interpolation Using Prelookup2/7, Interpolation Using Prelookup1/7
  ail_defl/1 -> WingRootPreLookup/1(ail_defl)
  WingRootPreLookup/4(Out4) -> Interpolation Using Prelookup6/4, Interpolation Using Prelookup5/4, Interpolation Using Prelookup4/4, Interpolation Using Prelookup3/4, Interpolation Using Prelookup2/4, Interpolation Using Prelookup1/4
  WingRootPreLookup/5(Out6) -> Interpolation Using Prelookup1/5, Interpolation Using Prelookup6/5, Interpolation Using Prelookup5/5, Interpolation Using Prelookup4/5, Interpolation Using Prelookup3/5, Interpolation Using Prelookup2/5
  Interpolation Using Prelookup1/1 -> CD/1
  WingRootPreLookup/6(Out7) -> Interpolation Using Prelookup6/6, Interpolation Using Prelookup5/6, Interpolation Using Prelookup4/6, Interpolation Using Prelookup3/6, Interpolation Using Prelookup2/6, Interpolation Using Prelookup1/6
  WingRootPreLookup/2(Out2) -> Interpolation Using Prelookup6/2, Interpolation Using Prelookup5/2, Interpolation Using Prelookup4/2, Interpolation Using Prelookup3/2, Interpolation Using Prelookup2/2, Interpolation Using Prelookup1/2
  DEP_J/1 -> WingRootPreLookup/4(DEP_J)
  V_node/1 -> WingRootPreLookup/3(V_node)
  alpha/1 -> WingRootPreLookup/2(alpha)
  Interpolation Using Prelookup2/1 -> CS/1
  Interpolation Using Prelookup3/1 -> CL/1
  Interpolation Using Prelookup4/1 -> CMx/1
  Interpolation Using Prelookup5/1 -> CMy/1
  Interpolation Using Prelookup6/1 -> CMz/1

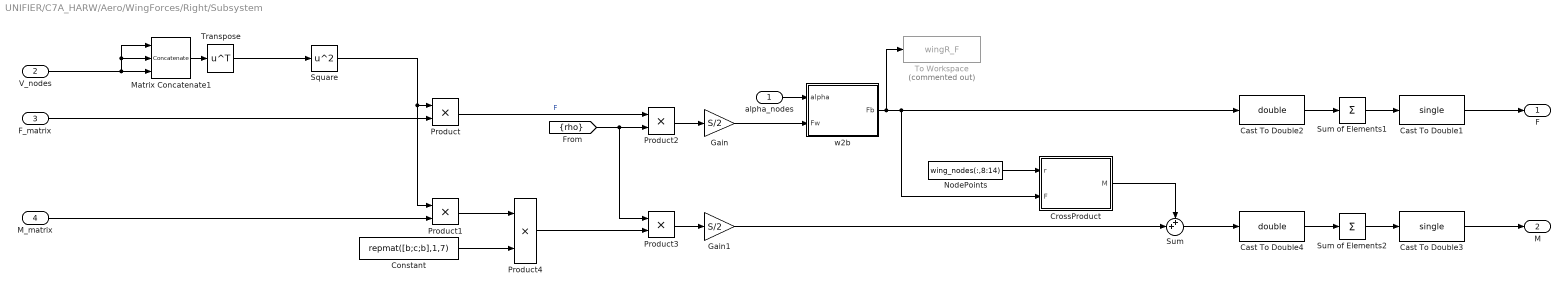
== system UNIFIER/C7A_HARW/Aero/WingForces/Right/Subsystem ==
  alpha_nodes : Inport
  V_nodes : Inport  Port=2
  F_matrix : Inport  Port=3
  M_matrix : Inport  Port=4
  Cast To Double1 : DataTypeConversion  OutDataTypeStr=single  SaturateOnIntegerOverflow=off  RndMeth=Floor
  Cast To Double2 : DataTypeConversion  OutDataTypeStr=double  SaturateOnIntegerOverflow=off  RndMeth=Floor
  Cast To Double3 : DataTypeConversion  OutDataTypeStr=single  SaturateOnIntegerOverflow=off  RndMeth=Floor
  Cast To Double4 : DataTypeConversion  OutDataTypeStr=double  SaturateOnIntegerOverflow=off  RndMeth=Floor
  Constant : Constant  Value=repmat([b;c;b],1,7)
  CrossProduct : Subsystem  TreatAsAtomicUnit=on
  Gain : Gain  Gain=S/2
  Gain1 : Gain  Gain=S/2
  Matrix Concatenate1 : Concatenate  NumInputs=3  Mode=Multidimensional array  ConcatenateDimension=2
  NodePoints : Constant  Value=wing_nodes(:,8:14)
  Product{,1..4} (5 alike) : Product
  Square : Math  Operator=square
  Sum : Sum  Inputs=++|
  Sum of Elements1 : Sum  Inputs=+  CollapseMode=Specified dimension  CollapseDim=2
  Sum of Elements2 : Sum  Inputs=+  CollapseMode=Specified dimension  CollapseDim=2
  To Workspace : ToWorkspace  Commented=on  VariableName=wingR_F  SaveFormat=Structure With Time  SampleTime=1/100
  Transpose : Math  Operator=transpose
  w2b : Subsystem  TreatAsAtomicUnit=on
  F : Outport
  M : Outport  Port=2
  wires:
  Product2/1 -> Gain/1
  F_matrix/1 -> Product/2
  [rho] -> Product3/1, Product2/2
  Product3/1 -> Gain1/1
  Constant/1 -> Product4/2
  Product4/1 -> Product3/2
  M_matrix/1 -> Product1/2
  Product1/1 -> Product4/1
  Gain1/1 -> Sum/2
  Product/1 -> Product2/1  "F"
  V_nodes/1 -> Matrix Concatenate1/1, Matrix Concatenate1/2, Matrix Concatenate1/3
  Transpose/1 -> Square/1
  Matrix Concatenate1/1 -> Transpose/1
  Square/1 -> Product1/1, Product/1
  NodePoints/1 -> CrossProduct/1(r)
  CrossProduct/1(M) -> Sum/1
  Cast To Double1/1 -> F/1
  Gain/1 -> w2b/2(Fw)
  alpha_nodes/1 -> w2b/1(alpha)
  Cast To Double2/1 -> Sum of Elements1/1
  Sum of Elements1/1 -> Cast To Double1/1
  Sum of Elements2/1 -> Cast To Double3/1
  Cast To Double4/1 -> Sum of Elements2/1
  Sum/1 -> Cast To Double4/1
  Cast To Double3/1 -> M/1
  w2b/1(Fb) -> To Workspace/1, Cast To Double2/1, CrossProduct/2(F)

== system UNIFIER/C7A_HARW/Aero/WingForces/Right/WingRootForces ==
  flap_defl : Inport
  alpha : Inport  Port=2
  V_node : Inport  Port=3
  DEP_J : Inport  Port=4
  Interpolation Using Prelookup1 : Interpolation_n-D  NumberOfTableDimensions=5  Table=dp_WING_root.CD  ExtrapMethod=Clip  ValidIndexMayReachLast=on  NumSelectionDims=1  InternalRulePriority=Speed  TableDataTypeStr=Inherit: Inherit from 'Table data'
      settings: InputPortMap=u0,u1,u2,u3,u4,u5,u6,u7,u8
  Interpolation Using Prelookup2 : Interpolation_n-D  NumberOfTableDimensions=5  Table=dp_WING_root.CS  ExtrapMethod=Clip  ValidIndexMayReachLast=on  NumSelectionDims=1  InternalRulePriority=Speed  TableDataTypeStr=Inherit: Inherit from 'Table data'
      settings: InputPortMap=u0,u1,u2,u3,u4,u5,u6,u7,u8
  Interpolation Using Prelookup3 : Interpolation_n-D  NumberOfTableDimensions=5  Table=dp_WING_root.CL  ExtrapMethod=Clip  ValidIndexMayReachLast=on  NumSelectionDims=1  InternalRulePriority=Speed  TableDataTypeStr=Inherit: Inherit from 'Table data'
      settings: InputPortMap=u0,u1,u2,u3,u4,u5,u6,u7,u8
  Interpolation Using Prelookup4 : Interpolation_n-D  NumberOfTableDimensions=5  Table=dp_WING_root.CMx  ExtrapMethod=Clip  ValidIndexMayReachLast=on  NumSelectionDims=1  InternalRulePriority=Speed  TableDataTypeStr=Inherit: Inherit from 'Table data'
      settings: InputPortMap=u0,u1,u2,u3,u4,u5,u6,u7,u8
  Interpolation Using Prelookup5 : Interpolation_n-D  NumberOfTableDimensions=5  Table=dp_WING_root.CMy  ExtrapMethod=Clip  ValidIndexMayReachLast=on  NumSelectionDims=1  InternalRulePriority=Speed  TableDataTypeStr=Inherit: Inherit from 'Table data'
      settings: InputPortMap=u0,u1,u2,u3,u4,u5,u6,u7,u8
  Interpolation Using Prelookup6 : Interpolation_n-D  NumberOfTableDimensions=5  Table=dp_WING_root.CMz  ExtrapMethod=Clip  ValidIndexMayReachLast=on  NumSelectionDims=1  InternalRulePriority=Speed  TableDataTypeStr=Inherit: Inherit from 'Table data'
      settings: InputPortMap=u0,u1,u2,u3,u4,u5,u6,u7,u8
  WingRootPreLookup : Subsystem
  CD : Outport
  CS : Outport  Port=2
  CL : Outport  Port=3
  CMx : Outport  Port=4
  CMy : Outport  Port=5
  CMz : Outport  Port=6
  wires:
  WingRootPreLookup/9(Out5) -> Interpolation Using Prelookup6/9, Interpolation Using Prelookup5/9, Interpolation Using Prelookup4/9, Interpolation Using Prelookup3/9, Interpolation Using Prelookup2/9, Interpolation Using Prelookup1/9
  WingRootPreLookup/3(Out3) -> Interpolation Using Prelookup6/3, Interpolation Using Prelookup5/3, Interpolation Using Prelookup4/3, Interpolation Using Prelookup3/3, Interpolation Using Prelookup2/3, Interpolation Using Prelookup1/3
  WingRootPreLookup/8(Out9) -> Interpolation Using Prelookup6/8, Interpolation Using Prelookup5/8, Interpolation Using Prelookup4/8, Interpolation Using Prelookup3/8, Interpolation Using Prelookup2/8, Interpolation Using Prelookup1/8
  WingRootPreLookup/1(Out1) -> Interpolation Using Prelookup6/1, Interpolation Using Prelookup5/1, Interpolation Using Prelookup4/1, Interpolation Using Prelookup3/1, Interpolation Using Prelookup2/1, Interpolation Using Prelookup1/1
  WingRootPreLookup/7(Out8) -> Interpolation Using Prelookup1/7, Interpolation Using Prelookup5/7, Interpolation Using Prelookup6/7, Interpolation Using Prelookup4/7, Interpolation Using Prelookup3/7, Interpolation Using Prelookup2/7
  flap_defl/1 -> WingRootPreLookup/1(flap_defl)
  WingRootPreLookup/4(Out4) -> Interpolation Using Prelookup6/4, Interpolation Using Prelookup5/4, Interpolation Using Prelookup4/4, Interpolation Using Prelookup3/4, Interpolation Using Prelookup2/4, Interpolation Using Prelookup1/4
  WingRootPreLookup/5(Out6) -> Interpolation Using Prelookup1/5, Interpolation Using Prelookup6/5, Interpolation Using Prelookup5/5, Interpolation Using Prelookup4/5, Interpolation Using Prelookup3/5, Interpolation Using Prelookup2/5
  Interpolation Using Prelookup1/1 -> CD/1
  WingRootPreLookup/6(Out7) -> Interpolation Using Prelookup6/6, Interpolation Using Prelookup5/6, Interpolation Using Prelookup4/6, Interpolation Using Prelookup3/6, Interpolation Using Prelookup2/6, Interpolation Using Prelookup1/6
  WingRootPreLookup/2(Out2) -> Interpolation Using Prelookup6/2, Interpolation Using Prelookup5/2, Interpolation Using Prelookup4/2, Interpolation Using Prelookup3/2, Interpolation Using Prelookup2/2, Interpolation Using Prelookup1/2
  DEP_J/1 -> WingRootPreLookup/4(DEP_J)
  V_node/1 -> WingRootPreLookup/3(V_node)
  alpha/1 -> WingRootPreLookup/2(alpha)
  Interpolation Using Prelookup2/1 -> CS/1
  Interpolation Using Prelookup3/1 -> CL/1
  Interpolation Using Prelookup4/1 -> CMx/1
  Interpolation Using Prelookup5/1 -> CMy/1
  Interpolation Using Prelookup6/1 -> CMz/1

== system UNIFIER/C7A_HARW/Aero/WingForces/Right/WingTipForces ==
  ail_defl : Inport
  alpha : Inport  Port=2
  V_node : Inport  Port=3
  DEP_J : Inport  Port=4
  Interpolation Using Prelookup1 : Interpolation_n-D  NumberOfTableDimensions=5  Table=dp_WING_tip.CD  ExtrapMethod=Clip  ValidIndexMayReachLast=on  NumSelectionDims=1  InternalRulePriority=Speed  TableDataTypeStr=Inherit: Inherit from 'Table data'
      settings: InputPortMap=u0,u1,u2,u3,u4,u5,u6,u7,u8
  Interpolation Using Prelookup2 : Interpolation_n-D  NumberOfTableDimensions=5  Table=dp_WING_tip.CS  ExtrapMethod=Clip  ValidIndexMayReachLast=on  NumSelectionDims=1  InternalRulePriority=Speed  TableDataTypeStr=Inherit: Inherit from 'Table data'
      settings: InputPortMap=u0,u1,u2,u3,u4,u5,u6,u7,u8
  Interpolation Using Prelookup3 : Interpolation_n-D  NumberOfTableDimensions=5  Table=dp_WING_tip.CL  ExtrapMethod=Clip  ValidIndexMayReachLast=on  NumSelectionDims=1  InternalRulePriority=Speed  TableDataTypeStr=Inherit: Inherit from 'Table data'
      settings: InputPortMap=u0,u1,u2,u3,u4,u5,u6,u7,u8
  Interpolation Using Prelookup4 : Interpolation_n-D  NumberOfTableDimensions=5  Table=dp_WING_tip.CMx  ExtrapMethod=Clip  ValidIndexMayReachLast=on  NumSelectionDims=1  InternalRulePriority=Speed  TableDataTypeStr=Inherit: Inherit from 'Table data'
      settings: InputPortMap=u0,u1,u2,u3,u4,u5,u6,u7,u8
  Interpolation Using Prelookup5 : Interpolation_n-D  NumberOfTableDimensions=5  Table=dp_WING_tip.CMy  ExtrapMethod=Clip  ValidIndexMayReachLast=on  NumSelectionDims=1  InternalRulePriority=Speed  TableDataTypeStr=Inherit: Inherit from 'Table data'
      settings: InputPortMap=u0,u1,u2,u3,u4,u5,u6,u7,u8
  Interpolation Using Prelookup6 : Interpolation_n-D  NumberOfTableDimensions=5  Table=dp_WING_tip.CMz  ExtrapMethod=Clip  ValidIndexMayReachLast=on  NumSelectionDims=1  InternalRulePriority=Speed  TableDataTypeStr=Inherit: Inherit from 'Table data'
      settings: InputPortMap=u0,u1,u2,u3,u4,u5,u6,u7,u8
  WingRootPreLookup : Subsystem
  CD : Outport
  CS : Outport  Port=2
  CL : Outport  Port=3
  CMx : Outport  Port=4
  CMy : Outport  Port=5
  CMz : Outport  Port=6
  wires:
  WingRootPreLookup/9(Out5) -> Interpolation Using Prelookup6/9, Interpolation Using Prelookup5/9, Interpolation Using Prelookup4/9, Interpolation Using Prelookup3/9, Interpolation Using Prelookup2/9, Interpolation Using Prelookup1/9
  WingRootPreLookup/3(Out3) -> Interpolation Using Prelookup6/3, Interpolation Using Prelookup5/3, Interpolation Using Prelookup4/3, Interpolation Using Prelookup3/3, Interpolation Using Prelookup2/3, Interpolation Using Prelookup1/3
  WingRootPreLookup/8(Out9) -> Interpolation Using Prelookup6/8, Interpolation Using Prelookup5/8, Interpolation Using Prelookup4/8, Interpolation Using Prelookup3/8, Interpolation Using Prelookup2/8, Interpolation Using Prelookup1/8
  WingRootPreLookup/1(Out1) -> Interpolation Using Prelookup6/1, Interpolation Using Prelookup5/1, Interpolation Using Prelookup4/1, Interpolation Using Prelookup3/1, Interpolation Using Prelookup2/1, Interpolation Using Prelookup1/1
  WingRootPreLookup/7(Out8) -> Interpolation Using Prelookup5/7, Interpolation Using Prelookup6/7, Interpolation Using Prelookup4/7, Interpolation Using Prelookup3/7, Interpolation Using Prelookup2/7, Interpolation Using Prelookup1/7
  ail_defl/1 -> WingRootPreLookup/1(ail_defl)
  WingRootPreLookup/4(Out4) -> Interpolation Using Prelookup6/4, Interpolation Using Prelookup5/4, Interpolation Using Prelookup4/4, Interpolation Using Prelookup3/4, Interpolation Using Prelookup2/4, Interpolation Using Prelookup1/4
  WingRootPreLookup/5(Out6) -> Interpolation Using Prelookup1/5, Interpolation Using Prelookup6/5, Interpolation Using Prelookup5/5, Interpolation Using Prelookup4/5, Interpolation Using Prelookup3/5, Interpolation Using Prelookup2/5
  Interpolation Using Prelookup1/1 -> CD/1
  WingRootPreLookup/6(Out7) -> Interpolation Using Prelookup6/6, Interpolation Using Prelookup5/6, Interpolation Using Prelookup4/6, Interpolation Using Prelookup3/6, Interpolation Using Prelookup2/6, Interpolation Using Prelookup1/6
  WingRootPreLookup/2(Out2) -> Interpolation Using Prelookup6/2, Interpolation Using Prelookup5/2, Interpolation Using Prelookup4/2, Interpolation Using Prelookup3/2, Interpolation Using Prelookup2/2, Interpolation Using Prelookup1/2
  DEP_J/1 -> WingRootPreLookup/4(DEP_J)
  V_node/1 -> WingRootPreLookup/3(V_node)
  alpha/1 -> WingRootPreLookup/2(alpha)
  Interpolation Using Prelookup2/1 -> CS/1
  Interpolation Using Prelookup3/1 -> CL/1
  Interpolation Using Prelookup4/1 -> CMx/1
  Interpolation Using Prelookup5/1 -> CMy/1
  Interpolation Using Prelookup6/1 -> CMz/1

== system UNIFIER/C7A_HARW/Subsystems/DEP/DEP/Controller ==
  actf : Inport
  Constant3 : Constant  Value=0
  Switch1 : Switch  Criteria=u2 > Threshold  Threshold=0.05  SaturateOnIntegerOverflow=off  InputSameDT=off
  T2rpm : Lookup_n-D  BreakpointsForDimension1=dp_DEP.rpm_lookup.V_vec  BreakpointsForDimension2=dp_DEP.rpm_lookup.T_vec  IndexSearchMethod=Linear search  BeginIndexSearchUsingPreviousIndexResult=on  Table=dp_DEP.rpm_lookup.rpm_gird  ExtrapMethod=Clip  InternalRulePriority=Speed  RndMeth=Simplest
      settings: InputPortMap=u0,u1
  actf2T : Gain  Gain=800
  rpm_cmd : Outport
  wires:
  actf2T/1 -> T2rpm/2
  Constant3/1 -> Switch1/3
  Switch1/1 -> rpm_cmd/1
  actf/1 -> Switch1/2, actf2T/1
  [V] -> T2rpm/1
  T2rpm/1 -> Switch1/1
